simulink model "program_simulink_1"  (R2024b)
settings: Solver=VariableStepAuto  StartTime=0.0  StopTime=3000  RelTol=1e-3
undefined symbols (not defined in the file): g, magnitude, rh, y0
settings Model: Creator=俞书阳  LastModifiedBy=user

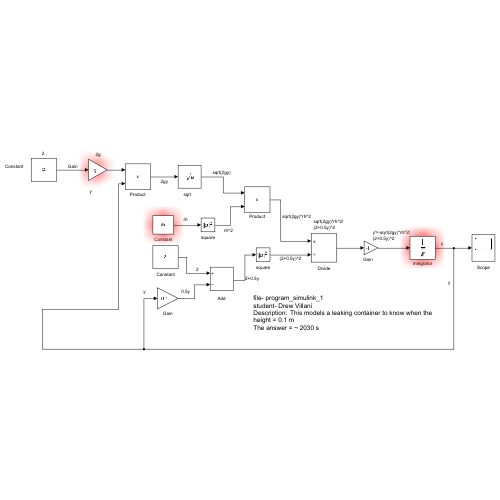
[thumbnail: Simulink's stored preview of the top-level diagram]
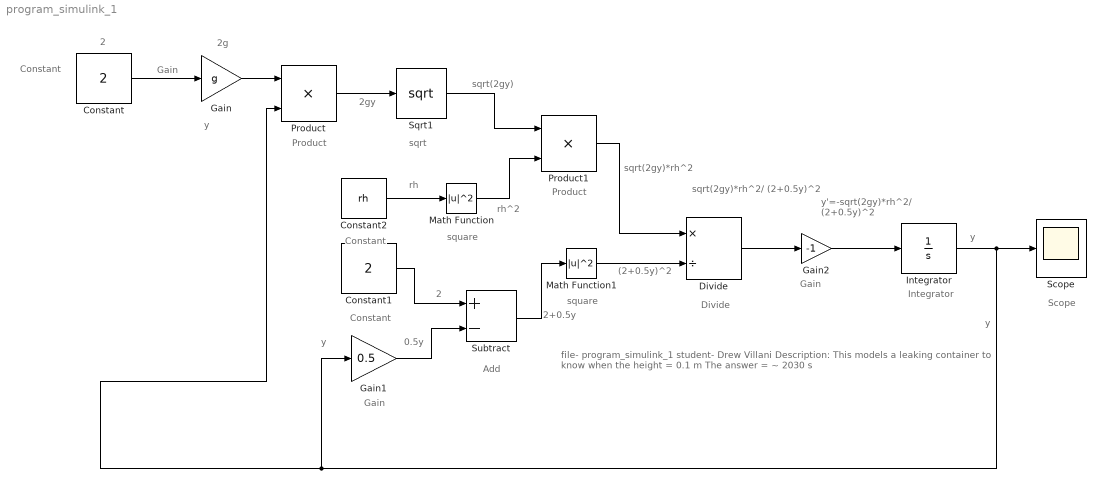
== system program_simulink_1 ==
  note: file- program_simulink_1
      | student- Drew Villani
      | Description: This models a leaking container to know when the height = 0.1 m
      | The answer = ~ 2030 s
  note: 0.5y
  note: 2
  note: y
  note: Scope
  note: Integrator
  note: Gain
  note: sqrt(2gy)*rh^2/
      | (2+0.5y)^2
  note: Divide
  note: Product
  note: (2+0.5y)^2
  note: square
  note: 2+0.5y
  note: Add
  note: Gain
  note: Constant
  note: y
  note: y
  note: rh^2
  note: square
  note: rh
  note: Constant
  note: sqrt(2gy)
  note: sqrt
  note: 2gy
  note: Product
  note: y
  note: 2g
  note: Gain
  note: 2
  note: Constant
  note: sqrt(2gy)*rh^2
  note: y'=-sqrt(2gy)*rh^2/
      | (2+0.5y)^2
  Constant : Constant  Value=2
  Constant1 : Constant  Value=2
  Constant2 : Constant  Value=rh
  Divide : Product  Inputs=*/
  Gain : Gain  Gain=g
  Gain1 : Gain  Gain=0.5
  Gain2 : Gain  Gain=-1
  Integrator : Integrator  InitialCondition=y0
  Math Function : Math  Operator=magnitude^2
  Math Function1 : Math  Operator=magnitude^2
  Product : Product
  Product1 : Product
  Scope : Scope
  Sqrt1 : Sqrt
  Subtract : Sum  Inputs=+-
  wires:
  Gain/1 -> Product/1
  Product/1 -> Sqrt1/1
  Constant/1 -> Gain/1
  Sqrt1/1 -> Product1/1
  Constant2/1 -> Math Function/1
  Math Function/1 -> Product1/2
  Product1/1 -> Divide/1
  Gain1/1 -> Subtract/2
  Constant1/1 -> Subtract/1
  Math Function1/1 -> Divide/2
  Subtract/1 -> Math Function1/1
  Divide/1 -> Gain2/1
  Integrator/1 -> Gain1/1, Product/2, Scope/1
  Gain2/1 -> Integrator/1
